simulink model "code_gen_HeadingHold"  (Simulink 7.5)
settings: Solver=FixedStepDiscrete  SolverMode=SingleTasking  StartTime=0.0  StopTime=10.0  FixedStep=0.01  RelTol=1e-3
InitFcn:
  | boat_constants
values from neighbouring files (symbols this model uses):
  figure8_waypoints = int32([ ... (first row only)    [boat_constants.m]
  OC2max = 49999    [boat_constants.m]    (also in simulation_constants.m)
  sampling_waypoints = int32([ ... (first row only)    [boat_constants.m]
  T_step = 0.01    [boat_constants.m]    (also in common.m)
  test_waypoints = int32([ ... (first row only)    [boat_constants.m]
undefined symbols (not defined in the file or in its folder): clearGpsData, clearSensorData, cpInitCommunications, DataEEInitAndClear, DataEEWrite, DiscIntNeverNeededParam, ecan1_buffered_transmit_matlab, ecan1_error_status_matlab, ecan1_init, ecan1_receive_matlab, getGpsData, getSensorData, Init_onlyOnce, Init_Reset, initCalibrationRange, initGps, processNewCommData, processNewGpsData, setHilMode, u1, u2, uart1EnqueueStateData, uart2EnqueueActuatorData, y1
libraries: simulink x85, dsPICdrivers x44, uSimLib x6, simulink_need_slupdate x4, aerolibconvert2 x2
(part 6 of 6)

== matlab function Sensor Inputs/Toggle1 ==
  data: u input double; y output double
function y = toggle(u)
%#eml

persistent pre_output;

% Initialize pre_output
if isempty(pre_output)
    pre_output = false;
end

% If we receive the toggle input, toggle
if u
    if pre_output
        pre_output = false;
    else
        pre_output = true;
    end
end

y = pre_output;

== matlab function Controller/Auto/Manual Switch/Rudder calibration controller/Run rudder for calibration ==
  data: trigger input double; step output double; rudder_port_limit input double; rudder_sb_limit input double; dir output double; throttle output double; rudder_position input double; mode output double
function [step, dir, throttle, mode] = calibrate(trigger, rudder_port_limit, rudder_sb_limit, rudder_position)
%#eml

% cal_state stores which state we're in. 0 indicates no calibration, 2 means
% calibrating the port limit, 1 means calibration the starboard limit
persistent cal_state direction run drive cal_mode
if isempty(cal_state)
    cal_state = uint8(0);
    direction = false;
    run = false;
    cal_mode = false;
    drive = true; % Drive is initialized to true here such that it will trigger a transition at the start and end of the calibration control code.
end

if trigger
    cal_mode = ~cal_mode;
end

mode = cal_mode;

if cal_state == 0 % Waiting for calibration trigger
    if trigger
        cal_state = uint8(6);
        drive = false;
    end
elseif cal_state == 6 % Initial calibration mode
    if ~cal_mode % Reset if calibration is disabled
        cal_state = uint8(0);
        run = false;
        drive = true;
    elseif rudder_sb_limit % If the starboard limit is active, go to port first
        cal_state = uint8(5);
        run = true;
        direction = true;
    else % Default to running to starboard first
        cal_state = uint8(4);
        run = true;
        direction = false;
    end
elseif cal_state == 5 % Calibrating the first limit (port)
    if ~cal_mode % Reset if calibration is disabled
        cal_state = uint8(0);
        run = false;
        drive = true;
    elseif rudder_port_limit % If we've hit the limit, we're done here
        cal_state = uint8(2);
        direction = false;
    end
elseif cal_state == 4 % Calibrating the first limit (starboard)
    if ~cal_mode % Reset if calibration is disabled
        cal_state = uint8(0);
        run = false;
        drive = true;
    elseif rudder_sb_limit % If we've hit the limit, we're done here
        cal_state = uint8(3);
        direction = true;
    end
elseif cal_state == 3 % Last limit calibration (port)
    if ~cal_mode % Reset if calibration is disabled
        cal_state = uint8(0);
        run = false;
        drive = true;
    elseif rudder_port_limit % If we've hit the port limit then we're done calibrating, so we recenter the rudder.
        cal_state = uint8(1);
        direction = false;
    end
elseif cal_state == 2 % Last limit calibration (starboard)
    if ~cal_mode % Reset if calibration is disabled
        cal_state = uint8(0);
        run = false;
        drive = true;
    elseif rudder_sb_limit % If we've hit the starboard limit then we're done calibrating, so we recenter the rudder.
        cal_state = uint8(1);
        direction = true;
    end
elseif cal_state == 1 % Center the rudder
    if ~cal_mode % Reset if calibration is disabled
        cal_state = uint8(0);
        run = false;
        drive = true;
    elseif abs(rudder_position) < 0.1 % If we're close to the center, stop commanding the rudder. Set to 0.1 to account for delay
        cal_state = uint8(0);
        run = false;
        drive = true;
        cal_mode = false;
    end
end

step = run;
dir = direction;
throttle = drive;
